simulink model "lorenz-simulink"  (R2022a)
settings: Solver=FixedStepAuto  StartTime=0.0  StopTime=25  FixedStep=0.001  RelTol=1e-3
settings Model: Creator=barrt  LastModifiedBy=barrt

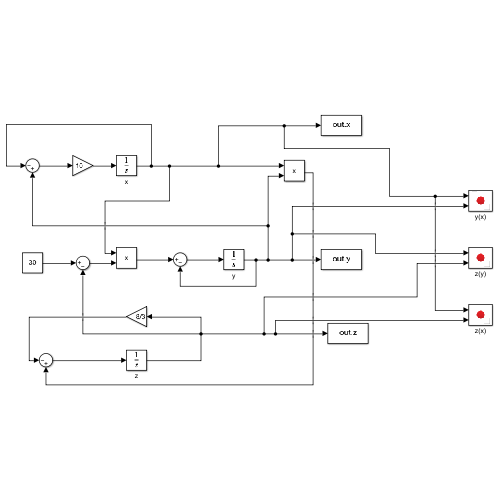
[thumbnail: Simulink's stored preview of the top-level diagram]
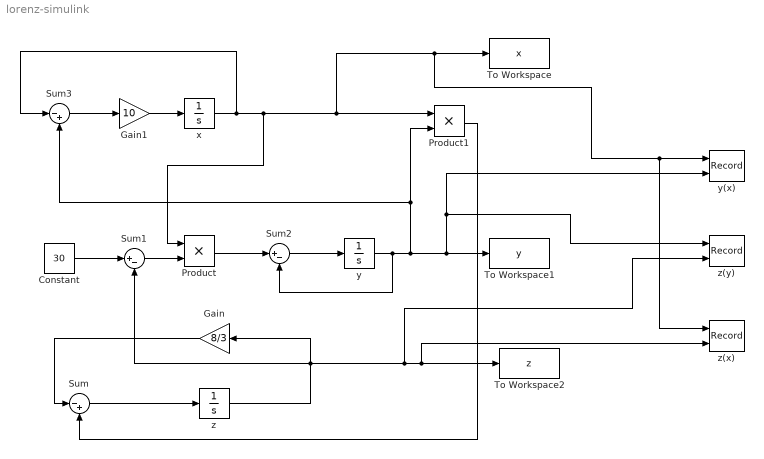
== system lorenz-simulink ==
  Constant : Constant  Value=30
  Gain : Gain  Gain=8/3
  Gain1 : Gain  Gain=10
  Product : Product
  Product1 : Product
  Sum : Sum  Inputs=|-+
  Sum1 : Sum  Inputs=|+-
  Sum2 : Sum  Inputs=|+-
  Sum3 : Sum  Inputs=|-+
  To Workspace : ToWorkspace  VariableName=x  SaveFormat=Timeseries  SampleTime=-1
  To Workspace1 : ToWorkspace  VariableName=y  SaveFormat=Timeseries  SampleTime=-1
  To Workspace2 : ToWorkspace  VariableName=z  SaveFormat=Timeseries  SampleTime=-1
  x : Integrator  InitialCondition=1
  y : Integrator  InitialCondition=1
  y(x) : Record  FileSettingsInternal="{\"entries\":[{\"content\":{\"excelSettings\":{\"content\":{},\"type\":\"Streamout.ExcelSettings\"}},\"type\":\"Streamout.FileSettingStorage\",\"uuid\":\"ef66f5b4-9747-4179-82e2-631585743150\"}],\"packageUris\":[\"http://schema.mathworks.com/mf0/streamout_blocks/R2020a\"],\"version\":\"1.0\"}"  Layout=[1 1]  SignalsInternal="{\"entries\":[{\"content\":{\"signals\":[{\"content\":{\"blockPath\":[\"untitled1/y(x)\"],\"channel\":[],\"dimensions\":[1],\"domain\":\"untitled1/y(x)\",\"lineColor\":\"#77ac30\",\"plots\":[],\"port\":1,\"sid\":[\"\"],\"signalID\":678,\"signalName\":\"x\"},\"type\":\"RecordBlkView.Signal\",\"uuid\":\"84917a2a-bbe2-48f7-bd10-169f3f3ae82a\"},{\"content\":{\"blockPath\":[\"untitled1/y(x)\"],\"channel\":[],\"dimensions\":[1],\"domain\":\"untitled1/y(x)\",\"lineColor\":\"#4dbeee\",\"plots\":[],\"port\":2,\"sid\":[\"\"],\"signalID\":682,\"signalName\":\"y\"},\"type\":\"RecordBlkView.Signal\",\"uuid\":\"8ff80d97-dd5b-42a3-82f1-5e98fa814d41\"}]},\"type\":\"RecordBlkView.InputSignals\",\"uuid\":\"5d19661e-52dc-48c4-bd58-6f340e3dbd91\"}],\"packageUris\":[\"http://schema.mathworks.com/mf0/streamout_blocks/R2020a\"],\"version\":\"1.0\"}"  VisualizationBindings="{\"xyplotplugin\":{\"info\":[{\"series\":[],\"subplotID\":1}]}}"  CompatibilityTag=XY
  z : Integrator  InitialCondition=1
  z(x) : Record  FileSettingsInternal="{\"entries\":[{\"content\":{\"excelSettings\":{\"content\":{},\"type\":\"Streamout.ExcelSettings\"}},\"type\":\"Streamout.FileSettingStorage\",\"uuid\":\"3a2009f5-ad20-4802-abaf-2a6bdb6587af\"}],\"packageUris\":[\"http://schema.mathworks.com/mf0/streamout_blocks/R2020a\"],\"version\":\"1.0\"}"  Layout=[1 1]  SignalsInternal="{\"entries\":[{\"content\":{\"signals\":[{\"content\":{\"blockPath\":[\"untitled1/z(x)\"],\"channel\":[],\"dimensions\":[1],\"domain\":\"untitled1/z(x)\",\"lineColor\":\"#a2142f\",\"plots\":[],\"port\":1,\"sid\":[\"\"],\"signalID\":686,\"signalName\":\"x\"},\"type\":\"RecordBlkView.Signal\",\"uuid\":\"4cb3b1a7-ae2e-49f6-b35d-81cf5174aa31\"},{\"content\":{\"blockPath\":[\"untitled1/z(x)\"],\"channel\":[],\"dimensions\":[1],\"domain\":\"untitled1/z(x)\",\"lineColor\":\"#139fff\",\"plots\":[],\"port\":2,\"sid\":[\"\"],\"signalID\":690,\"signalName\":\"z\"},\"type\":\"RecordBlkView.Signal\",\"uuid\":\"7219beb1-c581-4107-809a-961f9677b916\"}]},\"type\":\"RecordBlkView.InputSignals\",\"uuid\":\"d037b197-178a-4301-90ae-ddf2c226802c\"}],\"packageUris\":[\"http://schema.mathworks.com/mf0/streamout_blocks/R2020a\"],\"version\":\"1.0\"}"  VisualizationBindings="{\"xyplotplugin\":{\"info\":[{\"series\":[],\"subplotID\":1}]}}"  CompatibilityTag=XY
  z(y) : Record  FileSettingsInternal="{\"entries\":[{\"content\":{\"excelSettings\":{\"content\":{},\"type\":\"Streamout.ExcelSettings\"}},\"type\":\"Streamout.FileSettingStorage\",\"uuid\":\"f86f402a-50ec-4cfe-8e74-a88101df4387\"}],\"packageUris\":[\"http://schema.mathworks.com/mf0/streamout_blocks/R2020a\"],\"version\":\"1.0\"}"  Layout=[1 1]  SignalsInternal="{\"entries\":[{\"content\":{\"signals\":[{\"content\":{\"blockPath\":[\"untitled1/z(y)\"],\"channel\":[],\"dimensions\":[1],\"domain\":\"untitled1/z(y)\",\"lineColor\":\"#ff6929\",\"plots\":[],\"port\":1,\"sid\":[\"\"],\"signalID\":694,\"signalName\":\"y\"},\"type\":\"RecordBlkView.Signal\",\"uuid\":\"0b5130b6-c72f-4a90-87ea-a7eeac464065\"},{\"content\":{\"blockPath\":[\"untitled1/z(y)\"],\"channel\":[],\"dimensions\":[1],\"domain\":\"untitled1/z(y)\",\"lineColor\":\"#b746ff\",\"plots\":[],\"port\":2,\"sid\":[\"\"],\"signalID\":698,\"signalName\":\"z\"},\"type\":\"RecordBlkView.Signal\",\"uuid\":\"ad2a2e21-6257-404b-9541-81f01326f266\"}]},\"type\":\"RecordBlkView.InputSignals\",\"uuid\":\"7976e0c8-0c93-4bf2-be61-eacf9bec1b9c\"}],\"packageUris\":[\"http://schema.mathworks.com/mf0/streamout_blocks/R2020a\"],\"version\":\"1.0\"}"  VisualizationBindings="{\"xyplotplugin\":{\"info\":[{\"series\":[],\"subplotID\":1}]}}"  CompatibilityTag=XY
  wires:
  Sum1/1 -> Product/2
  Constant/1 -> Sum1/1
  Product/1 -> Sum2/1
  Sum2/1 -> y/1
  Sum3/1 -> Gain1/1
  Gain1/1 -> x/1
  y/1 -> Sum2/2, Sum3/2, Product1/2, z(y)/1, y(x)/2, To Workspace1/1
  Product1/1 -> Sum/2
  Gain/1 -> Sum/1
  Sum/1 -> z/1
  z/1 -> z(y)/2, z(x)/2, To Workspace2/1, Sum1/2, Gain/1
  x/1 -> Sum3/1, Product/1, z(x)/1, y(x)/1, To Workspace/1, Product1/1
